simulink library "halout"  (R2021b)
settings: Solver=VariableStepAuto  StartTime=0.0  StopTime=10.0  RelTol=1e-3
undefined symbols (not defined in the file): C_TASK_5MS_S, FALSE, KHAL_CAN1FD1APS3E2E_flg, KHAL_CAN1FD1APS3TxReq_flg, KHAL_CAN1FD1VCU2E2E_flg, KHAL_CAN1FD1VCU2TxReq_flg, KHAL_CAN1FD1VCU3E2E_flg, KHAL_CAN1FD1VCU3TxReq_flg, KHAL_CAN1TxReq_flg, KHAL_CAN1VMCFCM1E2E_flg, KHAL_CAN1VMCFCM1TxReq_flg, KHAL_CAN2TxReq_flg, KHAL_CAN3FD3VCU1toNIDECTxReq_flg, KHAL_CAN3FD3VCU1TxReq_flg, KHAL_CAN3FD3VCU2E2E_flg, KHAL_CAN3FD3VCU2toNIDECE2E_flg, KHAL_CAN3FD3VCU2toNIDECTxReq_flg, KHAL_CAN3FD3VCU2TxReq_flg, KHAL_CAN3TxReq_flg, KHAL_CAN4FD4CE1000E2E_flg, KHAL_CAN4FD4CE1000TxReq_flg, KHAL_CAN4TxReq_flg, KHAL_CAN5TxReq_flg, KHAL_CAN6FD6APS3E2E_flg, KHAL_CAN6FD6APS3TxReq_flg, KHAL_CAN6FD6VCU2E2E_flg, KHAL_CAN6FD6VCU2TxReq_flg, KHAL_CAN6TxReq_flg, ONE_INT, TRUE, ZERO_INT
libraries: FVT_lib x549, simulink x244
(part 15 of 27)

== system halout/HAL_OUT/CAN1/FD1_APS3_0x238/Byte_9 ==
  FDC_APS_Active_Sta : Inport
  FDC_APS_SpeedReq_Cmd : Inport  Port=2
  FDC_APS_VMCReqA_Cmd : Inport  Port=3
  FDC_RAPS_ErrLv1_Flg : Inport  Port=4
  FDC_VCU_RAPSErrLv2_Flg : Inport  Port=5
  BitwiseOR : simulink/Logic and Bit Operations/Bitwise Operator  logicop=OR  UseBitMask=off  NumInputPorts=5  BitMask=bin2dec('11011001')  BitMaskRealWorld=Stored Integer
  SignalPack : FVT_lib/hal/SignalPack  RightShiftCnt=0  BitMask=2^1-1  LeftShiftCnt=4
  SignalPack1 : FVT_lib/hal/SignalPack  RightShiftCnt=8  BitMask=2^4-1  LeftShiftCnt=0
  SignalPack2 : FVT_lib/hal/SignalPack  RightShiftCnt=0  BitMask=2^1-1  LeftShiftCnt=5
  SignalPack3 : FVT_lib/hal/SignalPack  RightShiftCnt=0  BitMask=2^1-1  LeftShiftCnt=6
  SignalPack4 : FVT_lib/hal/SignalPack  RightShiftCnt=0  BitMask=2^1-1  LeftShiftCnt=7
  UnitConverter{,1..2,4..9} (9 alike) : DataTypeConversion  OutDataTypeStr=uint8  RndMeth=Round
  UnitConverter3 : DataTypeConversion  OutDataTypeStr=uint16  RndMeth=Round
  convert_out : FVT_lib/hal/convert_out  gain=0.125  offset=0
  Byte_9 : Outport
  wires:
  BitwiseOR/1 -> Byte_9/1
  UnitConverter/1 -> BitwiseOR/1
  SignalPack/1 -> UnitConverter/1
  UnitConverter1/1 -> SignalPack/1
  FDC_APS_Active_Sta/1 -> UnitConverter1/1
  UnitConverter2/1 -> BitwiseOR/2
  SignalPack1/1 -> UnitConverter2/1
  UnitConverter3/1 -> SignalPack1/1
  convert_out/1 -> UnitConverter3/1
  FDC_APS_SpeedReq_Cmd/1 -> convert_out/1
  UnitConverter4/1 -> BitwiseOR/3
  SignalPack2/1 -> UnitConverter4/1
  UnitConverter5/1 -> SignalPack2/1
  FDC_APS_VMCReqA_Cmd/1 -> UnitConverter5/1
  UnitConverter6/1 -> BitwiseOR/4
  SignalPack3/1 -> UnitConverter6/1
  UnitConverter7/1 -> SignalPack3/1
  FDC_RAPS_ErrLv1_Flg/1 -> UnitConverter7/1
  UnitConverter8/1 -> BitwiseOR/5
  SignalPack4/1 -> UnitConverter8/1
  UnitConverter9/1 -> SignalPack4/1
  FDC_VCU_RAPSErrLv2_Flg/1 -> UnitConverter9/1

== system halout/HAL_OUT/CAN1/FD1_APS3_0x238/CAASSta ==
  CAASSta : Inport
  Data Type Conversion : DataTypeConversion  OutDataTypeStr=uint8  RndMeth=Round
  CAN1_CAAS_Sta : Outport
  wires:
  Data Type Conversion/1 -> CAN1_CAAS_Sta/1
  CAASSta/1 -> Data Type Conversion/1

== system halout/HAL_OUT/CAN1/FD1_APS3_0x238/CRC8_IfAction_Tx ==
  CAN_E2E_flg : Inport
  DataID1 : Inport  Port=2
  DataID2 : Inport  Port=3
  RawData : Inport  Port=4
  Data Type Conversion : DataTypeConversion  OutDataTypeStr=uint8
  If : If
  If Action Subsystem : Subsystem  TreatAsAtomicUnit=on
  If Action Subsystem1 : Subsystem  TreatAsAtomicUnit=on
  Merge : Merge
  CRC8 : Outport
  wires:
  If/2 -> If Action Subsystem/Action
  If/1 -> If Action Subsystem1/Action
  CAN_E2E_flg/1 -> [CAN_E2E_flg]
  DataID1/1 -> [DataID1]
  DataID2/1 -> [DataID2]
  RawData/1 -> [RawData]
  [CAN_E2E_flg] -> Data Type Conversion/1
  [DataID1] -> If Action Subsystem1/1(CAN_E2E_ID1)
  [DataID2] -> If Action Subsystem1/2(CAN_E2E_ID2)
  [RawData] -> If Action Subsystem1/3(Byte1)
  [RawData] -> If Action Subsystem/1(Byte1)
  If Action Subsystem1/1(CRC8_E2EResult) -> Merge/1
  If Action Subsystem/1(CRC8_Result) -> Merge/2
  Merge/1 -> CRC8/1
  Data Type Conversion/1 -> If/1

== system halout/HAL_OUT/CAN1/FD1_APS3_0x238/FDCAPSActiveSta ==
  FDCAPSActiveSta : Inport
  Data Type Conversion : DataTypeConversion  OutDataTypeStr=uint8  RndMeth=Round
  CAN1_FDC_APS_Active_Sta : Outport
  wires:
  Data Type Conversion/1 -> CAN1_FDC_APS_Active_Sta/1
  FDCAPSActiveSta/1 -> Data Type Conversion/1

== system halout/HAL_OUT/CAN1/FD1_APS3_0x238/FDCAPSCaasActiveSta ==
  FDCAPSCaasActiveSta : Inport
  Data Type Conversion : DataTypeConversion  OutDataTypeStr=uint8  RndMeth=Round
  CAN1_FDC_APS_CaasActive_Sta : Outport
  wires:
  Data Type Conversion/1 -> CAN1_FDC_APS_CaasActive_Sta/1
  FDCAPSCaasActiveSta/1 -> Data Type Conversion/1

== system halout/HAL_OUT/CAN1/FD1_APS3_0x238/FDCAPSCaasCtrlAvailSta ==
  FDCAPSCaasCtrlAvailSta : Inport
  Data Type Conversion : DataTypeConversion  OutDataTypeStr=uint8  RndMeth=Round
  CAN1_FDC_APS_CaasCtrlAvail_Sta : Outport
  wires:
  Data Type Conversion/1 -> CAN1_FDC_APS_CaasCtrlAvail_Sta/1
  FDCAPSCaasCtrlAvailSta/1 -> Data Type Conversion/1

== system halout/HAL_OUT/CAN1/FD1_APS3_0x238/FDCAPSCaasVMCReqACmd ==
  FDCAPSCaasVMCReqACmd : Inport
  Data Type Conversion : DataTypeConversion  OutDataTypeStr=uint8  RndMeth=Round
  CAN1_FDC_APS_CaasVMCReqA_Cmd : Outport
  wires:
  Data Type Conversion/1 -> CAN1_FDC_APS_CaasVMCReqA_Cmd/1
  FDCAPSCaasVMCReqACmd/1 -> Data Type Conversion/1

== system halout/HAL_OUT/CAN1/FD1_APS3_0x238/FDCAPSCtrlAvailSta ==
  FDCAPSCtrlAvailSta : Inport
  Data Type Conversion : DataTypeConversion  OutDataTypeStr=uint8  RndMeth=Round
  CAN1_FDC_APS_CtrlAvail_Sta : Outport
  wires:
  Data Type Conversion/1 -> CAN1_FDC_APS_CtrlAvail_Sta/1
  FDCAPSCtrlAvailSta/1 -> Data Type Conversion/1

== system halout/HAL_OUT/CAN1/FD1_APS3_0x238/FDCAPSShftPosnReqCmd ==
  FDCAPSShftPosnReqCmd : Inport
  Data Type Conversion : DataTypeConversion  OutDataTypeStr=uint8  RndMeth=Round
  CAN1_FDC_APS_ShftPosnReq_Cmd : Outport
  wires:
  Data Type Conversion/1 -> CAN1_FDC_APS_ShftPosnReq_Cmd/1
  FDCAPSShftPosnReqCmd/1 -> Data Type Conversion/1

== system halout/HAL_OUT/CAN1/FD1_APS3_0x238/FDCAPSSpeedReqCmd ==
  FDCAPSSpeedReqCmd : Inport
  Data Type Conversion : DataTypeConversion  OutDataTypeStr=uint16  RndMeth=Round
  convert_out : FVT_lib/hal/convert_out  gain=0.125  offset=0
  CAN1_FDC_APS_SpeedReq_Cmd : Outport
  wires:
  Data Type Conversion/1 -> CAN1_FDC_APS_SpeedReq_Cmd/1
  convert_out/1 -> Data Type Conversion/1
  FDCAPSSpeedReqCmd/1 -> convert_out/1

== system halout/HAL_OUT/CAN1/FD1_APS3_0x238/FDCAPSVMCReqACmd ==
  FDCAPSVMCReqACmd : Inport
  Data Type Conversion : DataTypeConversion  OutDataTypeStr=uint8  RndMeth=Round
  CAN1_FDC_APS_VMCReqA_Cmd : Outport
  wires:
  Data Type Conversion/1 -> CAN1_FDC_APS_VMCReqA_Cmd/1
  FDCAPSVMCReqACmd/1 -> Data Type Conversion/1

== system halout/HAL_OUT/CAN1/FD1_APS3_0x238/FDCRAPSBCMLampCmd ==
  FDCRAPSBCMLampCmd : Inport
  Data Type Conversion : DataTypeConversion  OutDataTypeStr=uint8  RndMeth=Round
  CAN1_FDC_RAPS_BCMLamp_Cmd : Outport
  wires:
  Data Type Conversion/1 -> CAN1_FDC_RAPS_BCMLamp_Cmd/1
  FDCRAPSBCMLampCmd/1 -> Data Type Conversion/1

== system halout/HAL_OUT/CAN1/FD1_APS3_0x238/FDCRAPSBCMLockReqCmd ==
  FDCRAPSBCMLockReqCmd : Inport
  Data Type Conversion : DataTypeConversion  OutDataTypeStr=uint8  RndMeth=Round
  CAN1_FDC_RAPS_BCMLockReq_Cmd : Outport
  wires:
  Data Type Conversion/1 -> CAN1_FDC_RAPS_BCMLockReq_Cmd/1
  FDCRAPSBCMLockReqCmd/1 -> Data Type Conversion/1

== system halout/HAL_OUT/CAN1/FD1_APS3_0x238/FDCRAPSErrLv1Flg ==
  FDCRAPSErrLv1Flg : Inport
  Data Type Conversion : DataTypeConversion  OutDataTypeStr=uint8  RndMeth=Round
  CAN1_FDC_RAPS_ErrLv1_Flg : Outport
  wires:
  Data Type Conversion/1 -> CAN1_FDC_RAPS_ErrLv1_Flg/1
  FDCRAPSErrLv1Flg/1 -> Data Type Conversion/1

== system halout/HAL_OUT/CAN1/FD1_APS3_0x238/FDCRAPSPwrReqAvailSta ==
  FDCRAPSPwrReqAvailSta : Inport
  Data Type Conversion : DataTypeConversion  OutDataTypeStr=uint8  RndMeth=Round
  CAN1_FDC_RAPS_PwrReqAvail_Sta : Outport
  wires:
  Data Type Conversion/1 -> CAN1_FDC_RAPS_PwrReqAvail_Sta/1
  FDCRAPSPwrReqAvailSta/1 -> Data Type Conversion/1

== system halout/HAL_OUT/CAN1/FD1_APS3_0x238/FDCRAPSPwrReqCmd ==
  FDCRAPSPwrReqCmd : Inport
  Data Type Conversion : DataTypeConversion  OutDataTypeStr=uint8  RndMeth=Round
  CAN1_FDC_RAPS_PwrReq_Cmd : Outport
  wires:
  Data Type Conversion/1 -> CAN1_FDC_RAPS_PwrReq_Cmd/1
  FDCRAPSPwrReqCmd/1 -> Data Type Conversion/1

== system halout/HAL_OUT/CAN1/FD1_APS3_0x238/FDCVCURAPSErrLv2Flg ==
  FDCVCURAPSErrLv2Flg : Inport
  Data Type Conversion : DataTypeConversion  OutDataTypeStr=uint8  RndMeth=Round
  CAN1_FDC_VCU_RAPSErrLv2_Flg : Outport
  wires:
  Data Type Conversion/1 -> CAN1_FDC_VCU_RAPSErrLv2_Flg/1
  FDCVCURAPSErrLv2Flg/1 -> Data Type Conversion/1

== system halout/HAL_OUT/CAN1/FD1_APS3_0x238/FDCVCURAPSErrLv3Flg ==
  FDCVCURAPSErrLv3Flg : Inport
  Data Type Conversion : DataTypeConversion  OutDataTypeStr=uint8  RndMeth=Round
  CAN1_FDC_VCU_RAPSErrLv3_Flg : Outport
  wires:
  Data Type Conversion/1 -> CAN1_FDC_VCU_RAPSErrLv3_Flg/1
  FDCVCURAPSErrLv3Flg/1 -> Data Type Conversion/1

== system halout/HAL_OUT/CAN1/FD1_APS3_0x238/FDCVMCAPSAngleTarget ==
  FDCVMCAPSAngleTarget : Inport
  Data Type Conversion : DataTypeConversion  OutDataTypeStr=uint16  RndMeth=Round
  convert_out : FVT_lib/hal/convert_out  gain=0.1  offset=-900
  CAN1_FDC_VMC_APS_Angle_Target : Outport
  wires:
  Data Type Conversion/1 -> CAN1_FDC_VMC_APS_Angle_Target/1
  convert_out/1 -> Data Type Conversion/1
  FDCVMCAPSAngleTarget/1 -> convert_out/1

== system halout/HAL_OUT/CAN1/FD1_APS3_0x238/FDCVMCAPSRqEPSCtrl ==
  FDCVMCAPSRqEPSCtrl : Inport
  Data Type Conversion : DataTypeConversion  OutDataTypeStr=uint8  RndMeth=Round
  CAN1_FDC_VMC_APS_Rq_EPS_Ctrl : Outport
  wires:
  Data Type Conversion/1 -> CAN1_FDC_VMC_APS_Rq_EPS_Ctrl/1
  FDCVMCAPSRqEPSCtrl/1 -> Data Type Conversion/1

== system halout/HAL_OUT/CAN1/FD1_APS3_0x238/FDCVMCAPSVRqEPSCtrl ==
  FDCVMCAPSVRqEPSCtrl : Inport
  Data Type Conversion : DataTypeConversion  OutDataTypeStr=uint8  RndMeth=Round
  CAN1_FDC_VMC_APS_V_Rq_EPS_Ctrl : Outport
  wires:
  Data Type Conversion/1 -> CAN1_FDC_VMC_APS_V_Rq_EPS_Ctrl/1
  FDCVMCAPSVRqEPSCtrl/1 -> Data Type Conversion/1

== system halout/HAL_OUT/CAN1/FD1_APS3_0x238/SPTGDet ==
  SPTGDet : Inport
  Data Type Conversion : DataTypeConversion  OutDataTypeStr=uint8  RndMeth=Round
  CAN1_SPTGDet : Outport
  wires:
  Data Type Conversion/1 -> CAN1_SPTGDet/1
  SPTGDet/1 -> Data Type Conversion/1

== system halout/HAL_OUT/CAN1/FD1_APS3_0x238/SPTGSta ==
  SPTGSta : Inport
  Data Type Conversion : DataTypeConversion  OutDataTypeStr=uint8  RndMeth=Round
  CAN1_SPTG_Sta : Outport
  wires:
  Data Type Conversion/1 -> CAN1_SPTG_Sta/1
  SPTGSta/1 -> Data Type Conversion/1

== system halout/HAL_OUT/CAN1/FD1_BCM1_0x216/AllDoorSW ==
  AllDoorSW : Inport
  Data Type Conversion : DataTypeConversion  OutDataTypeStr=uint8  RndMeth=Round
  CAN1_AllDoorSW : Outport
  wires:
  Data Type Conversion/1 -> CAN1_AllDoorSW/1
  AllDoorSW/1 -> Data Type Conversion/1

== system halout/HAL_OUT/CAN1/FD1_BCM1_0x216/AntiTheftSeatFold ==
  AntiTheftSeatFold : Inport
  Data Type Conversion : DataTypeConversion  OutDataTypeStr=uint8  RndMeth=Round
  CAN1_AntiTheftSeatFold : Outport
  wires:
  Data Type Conversion/1 -> CAN1_AntiTheftSeatFold/1
  AntiTheftSeatFold/1 -> Data Type Conversion/1

== system halout/HAL_OUT/CAN1/FD1_BCM1_0x216/AntitheftSta ==
  AntitheftSta : Inport
  Data Type Conversion : DataTypeConversion  OutDataTypeStr=uint8  RndMeth=Round
  CAN1_AntitheftSta : Outport
  wires:
  Data Type Conversion/1 -> CAN1_AntitheftSta/1
  AntitheftSta/1 -> Data Type Conversion/1

== system halout/HAL_OUT/CAN1/FD1_BCM1_0x216/BCMBuzzerReq ==
  BCMBuzzerReq : Inport
  Data Type Conversion : DataTypeConversion  OutDataTypeStr=uint8  RndMeth=Round
  CAN1_BCM_Buzzer_Req : Outport
  wires:
  Data Type Conversion/1 -> CAN1_BCM_Buzzer_Req/1
  BCMBuzzerReq/1 -> Data Type Conversion/1

== system halout/HAL_OUT/CAN1/FD1_BCM1_0x216/BCMDoorLockSta ==
  BCMDoorLockSta : Inport
  Data Type Conversion : DataTypeConversion  OutDataTypeStr=uint8  RndMeth=Round
  CAN1_BCM_DoorLock_Sta : Outport
  wires:
  Data Type Conversion/1 -> CAN1_BCM_DoorLock_Sta/1
  BCMDoorLockSta/1 -> Data Type Conversion/1

== system halout/HAL_OUT/CAN1/FD1_BCM1_0x216/BrakeLamp ==
  BrakeLamp : Inport
  Data Type Conversion : DataTypeConversion  OutDataTypeStr=uint8  RndMeth=Round
  CAN1_BrakeLamp : Outport
  wires:
  Data Type Conversion/1 -> CAN1_BrakeLamp/1
  BrakeLamp/1 -> Data Type Conversion/1

== system halout/HAL_OUT/CAN1/FD1_BCM1_0x216/CTDCtrl ==
  CTDCtrl : Inport
  Data Type Conversion : DataTypeConversion  OutDataTypeStr=uint8  RndMeth=Round
  CAN1_CTDCtrl : Outport
  wires:
  Data Type Conversion/1 -> CAN1_CTDCtrl/1
  CTDCtrl/1 -> Data Type Conversion/1

== system halout/HAL_OUT/CAN1/FD1_BCM1_0x216/CTDLockSW ==
  CTDLockSW : Inport
  Data Type Conversion : DataTypeConversion  OutDataTypeStr=uint8  RndMeth=Round
  CAN1_CTDLockSW : Outport
  wires:
  Data Type Conversion/1 -> CAN1_CTDLockSW/1
  CTDLockSW/1 -> Data Type Conversion/1

== system halout/HAL_OUT/CAN1/FD1_BCM1_0x216/CTDUnlockSW ==
  CTDUnlockSW : Inport
  Data Type Conversion : DataTypeConversion  OutDataTypeStr=uint8  RndMeth=Round
  CAN1_CTDUnlockSW : Outport
  wires:
  Data Type Conversion/1 -> CAN1_CTDUnlockSW/1
  CTDUnlockSW/1 -> Data Type Conversion/1

== system halout/HAL_OUT/CAN1/FD1_BCM1_0x216/CrashDetd ==
  CrashDetd : Inport
  Data Type Conversion : DataTypeConversion  OutDataTypeStr=uint8  RndMeth=Round
  CAN1_CrashDetd : Outport
  wires:
  Data Type Conversion/1 -> CAN1_CrashDetd/1
  CrashDetd/1 -> Data Type Conversion/1

== system halout/HAL_OUT/CAN1/FD1_BCM1_0x216/Dimmer ==
  Dimmer : Inport
  Data Type Conversion : DataTypeConversion  OutDataTypeStr=uint8  RndMeth=Round
  CAN1_Dimmer : Outport
  wires:
  Data Type Conversion/1 -> CAN1_Dimmer/1
  Dimmer/1 -> Data Type Conversion/1

== system halout/HAL_OUT/CAN1/FD1_BCM1_0x216/DimmerEN ==
  DimmerEN : Inport
  Data Type Conversion : DataTypeConversion  OutDataTypeStr=uint8  RndMeth=Round
  CAN1_DimmerEN : Outport
  wires:
  Data Type Conversion/1 -> CAN1_DimmerEN/1
  DimmerEN/1 -> Data Type Conversion/1

== system halout/HAL_OUT/CAN1/FD1_BCM1_0x216/DoorLockIND ==
  DoorLockIND : Inport
  Data Type Conversion : DataTypeConversion  OutDataTypeStr=uint8  RndMeth=Round
  CAN1_DoorLockIND : Outport
  wires:
  Data Type Conversion/1 -> CAN1_DoorLockIND/1
  DoorLockIND/1 -> Data Type Conversion/1

== system halout/HAL_OUT/CAN1/FD1_BCM1_0x216/DrDoorSW ==
  DrDoorSW : Inport
  Data Type Conversion : DataTypeConversion  OutDataTypeStr=uint8  RndMeth=Round
  CAN1_DrDoorSW : Outport
  wires:
  Data Type Conversion/1 -> CAN1_DrDoorSW/1
  DrDoorSW/1 -> Data Type Conversion/1

== system halout/HAL_OUT/CAN1/FD1_BCM1_0x216/FrChargingDoorCtrl ==
  FrChargingDoorCtrl : Inport
  Data Type Conversion : DataTypeConversion  OutDataTypeStr=uint8  RndMeth=Round
  CAN1_Fr_ChargingDoorCtrl : Outport
  wires:
  Data Type Conversion/1 -> CAN1_Fr_ChargingDoorCtrl/1
  FrChargingDoorCtrl/1 -> Data Type Conversion/1

== system halout/HAL_OUT/CAN1/FD1_BCM1_0x216/FrFogLamp ==
  FrFogLamp : Inport
  Data Type Conversion : DataTypeConversion  OutDataTypeStr=uint8  RndMeth=Round
  CAN1_Fr_FogLamp : Outport
  wires:
  Data Type Conversion/1 -> CAN1_Fr_FogLamp/1
  FrFogLamp/1 -> Data Type Conversion/1

== system halout/HAL_OUT/CAN1/FD1_BCM1_0x216/FrWiperH ==
  FrWiperH : Inport
  Data Type Conversion : DataTypeConversion  OutDataTypeStr=uint8  RndMeth=Round
  CAN1_Fr_Wiper_H : Outport
  wires:
  Data Type Conversion/1 -> CAN1_Fr_Wiper_H/1
  FrWiperH/1 -> Data Type Conversion/1

== system halout/HAL_OUT/CAN1/FD1_BCM1_0x216/FrWiperL ==
  FrWiperL : Inport
  Data Type Conversion : DataTypeConversion  OutDataTypeStr=uint8  RndMeth=Round
  CAN1_Fr_Wiper_L : Outport
  wires:
  Data Type Conversion/1 -> CAN1_Fr_Wiper_L/1
  FrWiperL/1 -> Data Type Conversion/1

== system halout/HAL_OUT/CAN1/FD1_BCM1_0x216/HBeam ==
  HBeam : Inport
  Data Type Conversion : DataTypeConversion  OutDataTypeStr=uint8  RndMeth=Round
  CAN1_H_Beam : Outport
  wires:
  Data Type Conversion/1 -> CAN1_H_Beam/1
  HBeam/1 -> Data Type Conversion/1

== system halout/HAL_OUT/CAN1/FD1_BCM1_0x216/HazardSW ==
  HazardSW : Inport
  Data Type Conversion : DataTypeConversion  OutDataTypeStr=uint8  RndMeth=Round
  CAN1_HazardSW : Outport
  wires:
  Data Type Conversion/1 -> CAN1_HazardSW/1
  HazardSW/1 -> Data Type Conversion/1

== system halout/HAL_OUT/CAN1/FD1_BCM1_0x216/HoodSW ==
  HoodSW : Inport
  Data Type Conversion : DataTypeConversion  OutDataTypeStr=uint8  RndMeth=Round
  CAN1_HoodSW : Outport
  wires:
  Data Type Conversion/1 -> CAN1_HoodSW/1
  HoodSW/1 -> Data Type Conversion/1

== system halout/HAL_OUT/CAN1/FD1_BCM1_0x216/HornCtrl ==
  HornCtrl : Inport
  Data Type Conversion : DataTypeConversion  OutDataTypeStr=uint8  RndMeth=Round
  CAN1_HornCtrl : Outport
  wires:
  Data Type Conversion/1 -> CAN1_HornCtrl/1
  HornCtrl/1 -> Data Type Conversion/1

== system halout/HAL_OUT/CAN1/FD1_BCM1_0x216/LAPMWdwEnable ==
  LAPMWdwEnable : Inport
  Data Type Conversion : DataTypeConversion  OutDataTypeStr=uint8  RndMeth=Round
  CAN1_L_APM_WdwEnable : Outport
  wires:
  Data Type Conversion/1 -> CAN1_L_APM_WdwEnable/1
  LAPMWdwEnable/1 -> Data Type Conversion/1

== system halout/HAL_OUT/CAN1/FD1_BCM1_0x216/LBSD ==
  LBSD : Inport
  Data Type Conversion : DataTypeConversion  OutDataTypeStr=uint8  RndMeth=Round
  CAN1_LBSD : Outport
  wires:
  Data Type Conversion/1 -> CAN1_LBSD/1
  LBSD/1 -> Data Type Conversion/1

== system halout/HAL_OUT/CAN1/FD1_BCM1_0x216/LBeam ==
  LBeam : Inport
  Data Type Conversion : DataTypeConversion  OutDataTypeStr=uint8  RndMeth=Round
  CAN1_L_Beam : Outport
  wires:
  Data Type Conversion/1 -> CAN1_L_Beam/1
  LBeam/1 -> Data Type Conversion/1

== system halout/HAL_OUT/CAN1/FD1_BCM1_0x216/LDRL ==
  LDRL : Inport
  Data Type Conversion : DataTypeConversion  OutDataTypeStr=uint8  RndMeth=Round
  CAN1_LDRL : Outport
  wires:
  Data Type Conversion/1 -> CAN1_LDRL/1
  LDRL/1 -> Data Type Conversion/1

== system halout/HAL_OUT/CAN1/FD1_BCM1_0x216/LTurnLP ==
  LTurnLP : Inport
  Data Type Conversion : DataTypeConversion  OutDataTypeStr=uint8  RndMeth=Round
  CAN1_LTurnLP : Outport
  wires:
  Data Type Conversion/1 -> CAN1_LTurnLP/1
  LTurnLP/1 -> Data Type Conversion/1

== system halout/HAL_OUT/CAN1/FD1_BCM1_0x216/LockSetting ==
  LockSetting : Inport
  Data Type Conversion : DataTypeConversion  OutDataTypeStr=uint8  RndMeth=Round
  CAN1_LockSetting : Outport
  wires:
  Data Type Conversion/1 -> CAN1_LockSetting/1
  LockSetting/1 -> Data Type Conversion/1

== system halout/HAL_OUT/CAN1/FD1_BCM1_0x216/MirrorCtrl ==
  MirrorCtrl : Inport
  Data Type Conversion : DataTypeConversion  OutDataTypeStr=uint8  RndMeth=Round
  CAN1_MirrorCtrl : Outport
  wires:
  Data Type Conversion/1 -> CAN1_MirrorCtrl/1
  MirrorCtrl/1 -> Data Type Conversion/1

== system halout/HAL_OUT/CAN1/FD1_BCM1_0x216/MirrorDefog ==
  MirrorDefog : Inport
  Data Type Conversion : DataTypeConversion  OutDataTypeStr=uint8  RndMeth=Round
  CAN1_MirrorDefog : Outport
  wires:
  Data Type Conversion/1 -> CAN1_MirrorDefog/1
  MirrorDefog/1 -> Data Type Conversion/1

== system halout/HAL_OUT/CAN1/FD1_BCM1_0x216/PosLamp ==
  PosLamp : Inport
  Data Type Conversion : DataTypeConversion  OutDataTypeStr=uint8  RndMeth=Round
  CAN1_PosLamp : Outport
  wires:
  Data Type Conversion/1 -> CAN1_PosLamp/1
  PosLamp/1 -> Data Type Conversion/1

== system halout/HAL_OUT/CAN1/FD1_BCM1_0x216/PsDoorSW ==
  PsDoorSW : Inport
  Data Type Conversion : DataTypeConversion  OutDataTypeStr=uint8  RndMeth=Round
  CAN1_PsDoorSW : Outport
  wires:
  Data Type Conversion/1 -> CAN1_PsDoorSW/1
  PsDoorSW/1 -> Data Type Conversion/1

== system halout/HAL_OUT/CAN1/FD1_BCM1_0x216/RBSD ==
  RBSD : Inport
  Data Type Conversion : DataTypeConversion  OutDataTypeStr=uint8  RndMeth=Round
  CAN1_RBSD : Outport
  wires:
  Data Type Conversion/1 -> CAN1_RBSD/1
  RBSD/1 -> Data Type Conversion/1

== system halout/HAL_OUT/CAN1/FD1_BCM1_0x216/RDRL ==
  RDRL : Inport
  Data Type Conversion : DataTypeConversion  OutDataTypeStr=uint8  RndMeth=Round
  CAN1_RDRL : Outport
  wires:
  Data Type Conversion/1 -> CAN1_RDRL/1
  RDRL/1 -> Data Type Conversion/1

== system halout/HAL_OUT/CAN1/FD1_BCM1_0x216/RLDoorSW ==
  RLDoorSW : Inport
  Data Type Conversion : DataTypeConversion  OutDataTypeStr=uint8  RndMeth=Round
  CAN1_RLDoorSW : Outport
  wires:
  Data Type Conversion/1 -> CAN1_RLDoorSW/1
  RLDoorSW/1 -> Data Type Conversion/1

== system halout/HAL_OUT/CAN1/FD1_BCM1_0x216/RRDoorSW ==
  RRDoorSW : Inport
  Data Type Conversion : DataTypeConversion  OutDataTypeStr=uint8  RndMeth=Round
  CAN1_RRDoorSW : Outport
  wires:
  Data Type Conversion/1 -> CAN1_RRDoorSW/1
  RRDoorSW/1 -> Data Type Conversion/1

== system halout/HAL_OUT/CAN1/FD1_BCM1_0x216/RTurnLP ==
  RTurnLP : Inport
  Data Type Conversion : DataTypeConversion  OutDataTypeStr=uint8  RndMeth=Round
  CAN1_RTurnLP : Outport
  wires:
  Data Type Conversion/1 -> CAN1_RTurnLP/1
  RTurnLP/1 -> Data Type Conversion/1

== system halout/HAL_OUT/CAN1/FD1_BCM1_0x216/ReverseLamp ==
  ReverseLamp : Inport
  Data Type Conversion : DataTypeConversion  OutDataTypeStr=uint8  RndMeth=Round
  CAN1_ReverseLamp : Outport
  wires:
  Data Type Conversion/1 -> CAN1_ReverseLamp/1
  ReverseLamp/1 -> Data Type Conversion/1

== system halout/HAL_OUT/CAN1/FD1_BCM1_0x216/RoomLampH ==
  RoomLampH : Inport
  Data Type Conversion : DataTypeConversion  OutDataTypeStr=uint8  RndMeth=Round
  CAN1_RoomLampH : Outport
  wires:
  Data Type Conversion/1 -> CAN1_RoomLampH/1
  RoomLampH/1 -> Data Type Conversion/1

== system halout/HAL_OUT/CAN1/FD1_BCM1_0x216/RoomLampL ==
  RoomLampL : Inport
  Data Type Conversion : DataTypeConversion  OutDataTypeStr=uint8  RndMeth=Round
  CAN1_RoomLampL : Outport
  wires:
  Data Type Conversion/1 -> CAN1_RoomLampL/1
  RoomLampL/1 -> Data Type Conversion/1

== system halout/HAL_OUT/CAN1/FD1_BCM1_0x216/RrChargingDoorCtrl ==
  RrChargingDoorCtrl : Inport
  Data Type Conversion : DataTypeConversion  OutDataTypeStr=uint8  RndMeth=Round
  CAN1_Rr_ChargingDoorCtrl : Outport
  wires:
  Data Type Conversion/1 -> CAN1_Rr_ChargingDoorCtrl/1
  RrChargingDoorCtrl/1 -> Data Type Conversion/1

== system halout/HAL_OUT/CAN1/FD1_BCM1_0x216/RrDefog ==
  RrDefog : Inport
  Data Type Conversion : DataTypeConversion  OutDataTypeStr=uint8  RndMeth=Round
  CAN1_Rr_Defog : Outport
  wires:
  Data Type Conversion/1 -> CAN1_Rr_Defog/1
  RrDefog/1 -> Data Type Conversion/1

== system halout/HAL_OUT/CAN1/FD1_BCM1_0x216/RrFogLamp ==
  RrFogLamp : Inport
  Data Type Conversion : DataTypeConversion  OutDataTypeStr=uint8  RndMeth=Round
  CAN1_Rr_FogLamp : Outport
  wires:
  Data Type Conversion/1 -> CAN1_Rr_FogLamp/1
  RrFogLamp/1 -> Data Type Conversion/1

== system halout/HAL_OUT/CAN1/FD1_BCM1_0x216/RrWiper ==
  RrWiper : Inport
  Data Type Conversion : DataTypeConversion  OutDataTypeStr=uint8  RndMeth=Round
  CAN1_Rr_Wiper : Outport
  wires:
  Data Type Conversion/1 -> CAN1_Rr_Wiper/1
  RrWiper/1 -> Data Type Conversion/1

== system halout/HAL_OUT/CAN1/FD1_BCM1_0x216/TailgateHDSW ==
  TailgateHDSW : Inport
  Data Type Conversion : DataTypeConversion  OutDataTypeStr=uint8  RndMeth=Round
  CAN1_TailgateHDSW : Outport
  wires:
  Data Type Conversion/1 -> CAN1_TailgateHDSW/1
  TailgateHDSW/1 -> Data Type Conversion/1

== system halout/HAL_OUT/CAN1/FD1_BCM1_0x216/TailgateRemote ==
  TailgateRemote : Inport
  Data Type Conversion : DataTypeConversion  OutDataTypeStr=uint8  RndMeth=Round
  CAN1_TailgateRemote : Outport
  wires:
  Data Type Conversion/1 -> CAN1_TailgateRemote/1
  TailgateRemote/1 -> Data Type Conversion/1

== system halout/HAL_OUT/CAN1/FD1_BCM1_0x216/TailgateSW ==
  TailgateSW : Inport
  Data Type Conversion : DataTypeConversion  OutDataTypeStr=uint8  RndMeth=Round
  CAN1_Tailgate_SW : Outport
  wires:
  Data Type Conversion/1 -> CAN1_Tailgate_SW/1
  TailgateSW/1 -> Data Type Conversion/1

== system halout/HAL_OUT/CAN1/FD1_BCM1_0x216/TrunkRel ==
  TrunkRel : Inport
  Data Type Conversion : DataTypeConversion  OutDataTypeStr=uint8  RndMeth=Round
  CAN1_TrunkRel : Outport
  wires:
  Data Type Conversion/1 -> CAN1_TrunkRel/1
  TrunkRel/1 -> Data Type Conversion/1

== system halout/HAL_OUT/CAN1/FD1_BCM1_0x216/WasherCtrl ==
  WasherCtrl : Inport
  Data Type Conversion : DataTypeConversion  OutDataTypeStr=uint8  RndMeth=Round
  CAN1_WasherCtrl : Outport
  wires:
  Data Type Conversion/1 -> CAN1_WasherCtrl/1
  WasherCtrl/1 -> Data Type Conversion/1

== system halout/HAL_OUT/CAN1/FD1_BCM1_0x216/WiperFixMode ==
  WiperFixMode : Inport
  Data Type Conversion : DataTypeConversion  OutDataTypeStr=uint8  RndMeth=Round
  CAN1_WiperFixMode : Outport
  wires:
  Data Type Conversion/1 -> CAN1_WiperFixMode/1
  WiperFixMode/1 -> Data Type Conversion/1

== system halout/HAL_OUT/CAN1/FD1_THCM1_0x182/BatteryMode ==
  BatteryMode : Inport
  Data Type Conversion : DataTypeConversion  OutDataTypeStr=uint8  RndMeth=Round
  CAN1_BatteryMode : Outport
  wires:
  Data Type Conversion/1 -> CAN1_BatteryMode/1
  BatteryMode/1 -> Data Type Conversion/1

== system halout/HAL_OUT/CAN1/FD1_THCM1_0x182/CCUACLampSts ==
  CCUACLampSts : Inport
  Data Type Conversion : DataTypeConversion  OutDataTypeStr=uint8  RndMeth=Round
  CAN1_CCU_ACLampSts : Outport
  wires:
  Data Type Conversion/1 -> CAN1_CCU_ACLampSts/1
  CCUACLampSts/1 -> Data Type Conversion/1

== system halout/HAL_OUT/CAN1/FD1_THCM1_0x182/CCUACMaxLampSts ==
  CCUACMaxLampSts : Inport
  Data Type Conversion : DataTypeConversion  OutDataTypeStr=uint8  RndMeth=Round
  CAN1_CCU_ACMaxLampSts : Outport
  wires:
  Data Type Conversion/1 -> CAN1_CCU_ACMaxLampSts/1
  CCUACMaxLampSts/1 -> Data Type Conversion/1

== system halout/HAL_OUT/CAN1/FD1_THCM1_0x182/CCUAutoLampSts ==
  CCUAutoLampSts : Inport
  Data Type Conversion : DataTypeConversion  OutDataTypeStr=uint8  RndMeth=Round
  CAN1_CCU_AutoLampSts : Outport
  wires:
  Data Type Conversion/1 -> CAN1_CCU_AutoLampSts/1
  CCUAutoLampSts/1 -> Data Type Conversion/1

== system halout/HAL_OUT/CAN1/FD1_THCM1_0x182/CCUAutoMidLampSts ==
  CCUAutoMidLampSts : Inport
  Data Type Conversion : DataTypeConversion  OutDataTypeStr=uint8  RndMeth=Round
  CAN1_CCU_AutoMidLampSts : Outport
  wires:
  Data Type Conversion/1 -> CAN1_CCU_AutoMidLampSts/1
  CCUAutoMidLampSts/1 -> Data Type Conversion/1

== system halout/HAL_OUT/CAN1/FD1_THCM1_0x182/CCUDispalyRequest ==
  CCUDispalyRequest : Inport
  Data Type Conversion : DataTypeConversion  OutDataTypeStr=uint8  RndMeth=Round
  CAN1_CCU_Dispaly_Request : Outport
  wires:
  Data Type Conversion/1 -> CAN1_CCU_Dispaly_Request/1
  CCUDispalyRequest/1 -> Data Type Conversion/1

== system halout/HAL_OUT/CAN1/FD1_THCM1_0x182/CCUEcoSts ==
  CCUEcoSts : Inport
  Data Type Conversion : DataTypeConversion  OutDataTypeStr=uint8  RndMeth=Round
  CAN1_CCU_EcoSts : Outport
  wires:
  Data Type Conversion/1 -> CAN1_CCU_EcoSts/1
  CCUEcoSts/1 -> Data Type Conversion/1

== system halout/HAL_OUT/CAN1/FD1_THCM1_0x182/CCUFrtOnOffLampSts ==
  CCUFrtOnOffLampSts : Inport
  Data Type Conversion : DataTypeConversion  OutDataTypeStr=uint8  RndMeth=Round
  CAN1_CCU_FrtOnOffLampSts : Outport
  wires:
  Data Type Conversion/1 -> CAN1_CCU_FrtOnOffLampSts/1
  CCUFrtOnOffLampSts/1 -> Data Type Conversion/1

== system halout/HAL_OUT/CAN1/FD1_THCM1_0x182/CCUHEATMaxLampSts ==
  CCUHEATMaxLampSts : Inport
  Data Type Conversion : DataTypeConversion  OutDataTypeStr=uint8  RndMeth=Round
  CAN1_CCU_HEATMaxLampSts : Outport
  wires:
  Data Type Conversion/1 -> CAN1_CCU_HEATMaxLampSts/1
  CCUHEATMaxLampSts/1 -> Data Type Conversion/1

== system halout/HAL_OUT/CAN1/FD1_THCM1_0x182/CCURrOnOffLampSts ==
  CCURrOnOffLampSts : Inport
  Data Type Conversion : DataTypeConversion  OutDataTypeStr=uint8  RndMeth=Round
  CAN1_CCU_RrOnOffLampSts : Outport
  wires:
  Data Type Conversion/1 -> CAN1_CCU_RrOnOffLampSts/1
  CCURrOnOffLampSts/1 -> Data Type Conversion/1

== system halout/HAL_OUT/CAN1/FD1_THCM1_0x182/CCUSyncLampSts ==
  CCUSyncLampSts : Inport
  Data Type Conversion : DataTypeConversion  OutDataTypeStr=uint8  RndMeth=Round
  CAN1_CCU_SyncLampSts : Outport
  wires:
  Data Type Conversion/1 -> CAN1_CCU_SyncLampSts/1
  CCUSyncLampSts/1 -> Data Type Conversion/1

== system halout/HAL_OUT/CAN1/FD1_THCM1_0x182/CabinMode ==
  CabinMode : Inport
  Data Type Conversion : DataTypeConversion  OutDataTypeStr=uint8  RndMeth=Round
  CAN1_CabinMode : Outport
  wires:
  Data Type Conversion/1 -> CAN1_CabinMode/1
  CabinMode/1 -> Data Type Conversion/1

== system halout/HAL_OUT/CAN1/FD1_THCM1_0x182/EDriveMode ==
  EDriveMode : Inport
  Data Type Conversion : DataTypeConversion  OutDataTypeStr=uint8  RndMeth=Round
  CAN1_EDriveMode : Outport
  wires:
  Data Type Conversion/1 -> CAN1_EDriveMode/1
  EDriveMode/1 -> Data Type Conversion/1

== system halout/HAL_OUT/CAN1/FD1_THCM1_0x182/FDAGSCmd ==
  FDAGSCmd : Inport
  Data Type Conversion : DataTypeConversion  OutDataTypeStr=uint8  RndMeth=Round
  CAN1_FD_AGS_Cmd : Outport
  wires:
  Data Type Conversion/1 -> CAN1_FD_AGS_Cmd/1
  FDAGSCmd/1 -> Data Type Conversion/1

== system halout/HAL_OUT/CAN1/FD1_THCM1_0x182/FDRecyAutoCmd ==
  FDRecyAutoCmd : Inport
  Data Type Conversion : DataTypeConversion  OutDataTypeStr=uint8  RndMeth=Round
  CAN1_FD_RecyAuto_Cmd : Outport
  wires:
  Data Type Conversion/1 -> CAN1_FD_RecyAuto_Cmd/1
  FDRecyAutoCmd/1 -> Data Type Conversion/1

== system halout/HAL_OUT/CAN1/FD1_THCM1_0x182/FrCoolantflow ==
  FrCoolantflow : Inport
  Data Type Conversion : DataTypeConversion  OutDataTypeStr=uint8  RndMeth=Round
  convert_out : FVT_lib/hal/convert_out  gain=0.25  offset=0
  CAN1_Fr_Coolantflow : Outport
  wires:
  Data Type Conversion/1 -> CAN1_Fr_Coolantflow/1
  convert_out/1 -> Data Type Conversion/1
  FrCoolantflow/1 -> convert_out/1

== system halout/HAL_OUT/CAN1/FD1_THCM1_0x182/FrCoolanttemp ==
  FrCoolanttemp : Inport
  Data Type Conversion : DataTypeConversion  OutDataTypeStr=uint16  RndMeth=Round
  convert_out : FVT_lib/hal/convert_out  gain=1  offset=-40
  CAN1_Fr_Coolanttemp : Outport
  wires:
  Data Type Conversion/1 -> CAN1_Fr_Coolanttemp/1
  convert_out/1 -> Data Type Conversion/1
  FrCoolanttemp/1 -> convert_out/1

== system halout/HAL_OUT/CAN1/FD1_THCM1_0x182/HPThermalRecoveryReq ==
  HPThermalRecoveryReq : Inport
  Data Type Conversion : DataTypeConversion  OutDataTypeStr=uint8  RndMeth=Round
  CAN1_HPThermalRecoveryReq : Outport
  wires:
  Data Type Conversion/1 -> CAN1_HPThermalRecoveryReq/1
  HPThermalRecoveryReq/1 -> Data Type Conversion/1

== system halout/HAL_OUT/CAN1/FD1_THCM1_0x182/RrCoolantflow ==
  RrCoolantflow : Inport
  Data Type Conversion : DataTypeConversion  OutDataTypeStr=uint8  RndMeth=Round
  convert_out : FVT_lib/hal/convert_out  gain=0.25  offset=0
  CAN1_Rr_Coolantflow : Outport
  wires:
  Data Type Conversion/1 -> CAN1_Rr_Coolantflow/1
  convert_out/1 -> Data Type Conversion/1
  RrCoolantflow/1 -> convert_out/1

== system halout/HAL_OUT/CAN1/FD1_THCM1_0x182/RrCoolanttemp ==
  RrCoolanttemp : Inport
  Data Type Conversion : DataTypeConversion  OutDataTypeStr=uint16  RndMeth=Round
  convert_out : FVT_lib/hal/convert_out  gain=1  offset=-40
  CAN1_Rr_Coolanttemp : Outport
  wires:
  Data Type Conversion/1 -> CAN1_Rr_Coolanttemp/1
  convert_out/1 -> Data Type Conversion/1
  RrCoolanttemp/1 -> convert_out/1

== system halout/HAL_OUT/CAN1/FD1_THCM1_0x182/sigAirIntenZon1St ==
  sigAirIntenZon1St : Inport
  Data Type Conversion : DataTypeConversion  OutDataTypeStr=uint8  RndMeth=Round
  CAN1_sigAirIntenZon1St : Outport
  wires:
  Data Type Conversion/1 -> CAN1_sigAirIntenZon1St/1
  sigAirIntenZon1St/1 -> Data Type Conversion/1

== system halout/HAL_OUT/CAN1/FD1_THCM1_0x182/sigAirIntenZon3St ==
  sigAirIntenZon3St : Inport
  Data Type Conversion : DataTypeConversion  OutDataTypeStr=uint8  RndMeth=Round
  CAN1_sigAirIntenZon3St : Outport
  wires:
  Data Type Conversion/1 -> CAN1_sigAirIntenZon3St/1
  sigAirIntenZon3St/1 -> Data Type Conversion/1

== system halout/HAL_OUT/CAN1/FD1_THCM1_0x182/sigAmbAirT ==
  sigAmbAirT : Inport
  Data Type Conversion : DataTypeConversion  OutDataTypeStr=uint8  RndMeth=Round
  convert_out : FVT_lib/hal/convert_out  gain=0.5  offset=-40
  CAN1_sigAmbAirT : Outport
  wires:
  Data Type Conversion/1 -> CAN1_sigAmbAirT/1
  convert_out/1 -> Data Type Conversion/1
  sigAmbAirT/1 -> convert_out/1

== system halout/HAL_OUT/CAN1/FD1_THCM1_0x182/sigCbnAirT ==
  sigCbnAirT : Inport
  Data Type Conversion : DataTypeConversion  OutDataTypeStr=uint8  RndMeth=Round
  convert_out : FVT_lib/hal/convert_out  gain=0.5  offset=-40
  CAN1_sigCbnAirT : Outport
  wires:
  Data Type Conversion/1 -> CAN1_sigCbnAirT/1
  convert_out/1 -> Data Type Conversion/1
  sigCbnAirT/1 -> convert_out/1

== system halout/HAL_OUT/CAN1/FD1_THCM1_0x182/sigCbnPTCPwrAct ==
  sigCbnPTCPwrAct : Inport
  Data Type Conversion : DataTypeConversion  OutDataTypeStr=uint8  RndMeth=Round
  convert_out : FVT_lib/hal/convert_out  gain=50  offset=0
  CAN1_sigCbnPTCPwrAct : Outport
  wires:
  Data Type Conversion/1 -> CAN1_sigCbnPTCPwrAct/1
  convert_out/1 -> Data Type Conversion/1
  sigCbnPTCPwrAct/1 -> convert_out/1

== system halout/HAL_OUT/CAN1/FD1_THCM1_0x182/sigCbnSolarLeft ==
  sigCbnSolarLeft : Inport
  Data Type Conversion : DataTypeConversion  OutDataTypeStr=uint8  RndMeth=Round
  convert_out : FVT_lib/hal/convert_out  gain=5  offset=0
  CAN1_sigCbnSolarLeft : Outport
  wires:
  Data Type Conversion/1 -> CAN1_sigCbnSolarLeft/1
  convert_out/1 -> Data Type Conversion/1
  sigCbnSolarLeft/1 -> convert_out/1

== system halout/HAL_OUT/CAN1/FD1_THCM1_0x182/sigCbnSolarRight ==
  sigCbnSolarRight : Inport
  Data Type Conversion : DataTypeConversion  OutDataTypeStr=uint8  RndMeth=Round
  convert_out : FVT_lib/hal/convert_out  gain=5  offset=0
  CAN1_sigCbnSolarRight : Outport
  wires:
  Data Type Conversion/1 -> CAN1_sigCbnSolarRight/1
  convert_out/1 -> Data Type Conversion/1
  sigCbnSolarRight/1 -> convert_out/1

== system halout/HAL_OUT/CAN1/FD1_THCM1_0x182/sigClmtCmprPwrAct ==
  sigClmtCmprPwrAct : Inport
  Data Type Conversion : DataTypeConversion  OutDataTypeStr=uint8  RndMeth=Round
  convert_out : FVT_lib/hal/convert_out  gain=50  offset=0
  CAN1_sigClmtCmprPwrAct : Outport
  wires:
  Data Type Conversion/1 -> CAN1_sigClmtCmprPwrAct/1
  convert_out/1 -> Data Type Conversion/1
  sigClmtCmprPwrAct/1 -> convert_out/1

== system halout/HAL_OUT/CAN1/FD1_THCM1_0x182/sigClntTHvBattOut ==
  sigClntTHvBattOut : Inport
  Data Type Conversion : DataTypeConversion  OutDataTypeStr=uint8  RndMeth=Round
  convert_out : FVT_lib/hal/convert_out  gain=0.5  offset=-40
  CAN1_sigClntTHvBattOut : Outport
  wires:
  Data Type Conversion/1 -> CAN1_sigClntTHvBattOut/1
  convert_out/1 -> Data Type Conversion/1
  sigClntTHvBattOut/1 -> convert_out/1

== system halout/HAL_OUT/CAN1/FD1_THCM1_0x182/sigDfrstSt ==
  sigDfrstSt : Inport
  Data Type Conversion : DataTypeConversion  OutDataTypeStr=uint8  RndMeth=Round
  CAN1_sigDfrstSt : Outport
  wires:
  Data Type Conversion/1 -> CAN1_sigDfrstSt/1
  sigDfrstSt/1 -> Data Type Conversion/1

== system halout/HAL_OUT/CAN1/FD1_THCM1_0x182/sigHvacSt ==
  sigHvacSt : Inport
  Data Type Conversion : DataTypeConversion  OutDataTypeStr=uint8  RndMeth=Round
  CAN1_sigHvacSt : Outport
  wires:
  Data Type Conversion/1 -> CAN1_sigHvacSt/1
  sigHvacSt/1 -> Data Type Conversion/1

== system halout/HAL_OUT/CAN1/FD1_THCM1_0x182/sigRecircSt ==
  sigRecircSt : Inport
  Data Type Conversion : DataTypeConversion  OutDataTypeStr=uint8  RndMeth=Round
  CAN1_sigRecircSt : Outport
  wires:
  Data Type Conversion/1 -> CAN1_sigRecircSt/1
  sigRecircSt/1 -> Data Type Conversion/1

== system halout/HAL_OUT/CAN1/FD1_THCM1_0x182/sigSetTempZon1St ==
  sigSetTempZon1St : Inport
  Data Type Conversion : DataTypeConversion  OutDataTypeStr=uint8  RndMeth=Round
  convert_out : FVT_lib/hal/convert_out  gain=0.5  offset=17
  CAN1_sigSetTempZon1St : Outport
  wires:
  Data Type Conversion/1 -> CAN1_sigSetTempZon1St/1
  convert_out/1 -> Data Type Conversion/1
  sigSetTempZon1St/1 -> convert_out/1

== system halout/HAL_OUT/CAN1/FD1_THCM1_0x182/sigSetTempZon2St ==
  sigSetTempZon2St : Inport
  Data Type Conversion : DataTypeConversion  OutDataTypeStr=uint8  RndMeth=Round
  convert_out : FVT_lib/hal/convert_out  gain=0.5  offset=17
  CAN1_sigSetTempZon2St : Outport
  wires:
  Data Type Conversion/1 -> CAN1_sigSetTempZon2St/1
  convert_out/1 -> Data Type Conversion/1
  sigSetTempZon2St/1 -> convert_out/1

== system halout/HAL_OUT/CAN1/FD1_THCM1_0x182/sigSetTempZon3St ==
  sigSetTempZon3St : Inport
  Data Type Conversion : DataTypeConversion  OutDataTypeStr=uint8  RndMeth=Round
  convert_out : FVT_lib/hal/convert_out  gain=0.5  offset=17
  CAN1_sigSetTempZon3St : Outport
  wires:
  Data Type Conversion/1 -> CAN1_sigSetTempZon3St/1
  convert_out/1 -> Data Type Conversion/1
  sigSetTempZon3St/1 -> convert_out/1

== system halout/HAL_OUT/CAN1/FD1_THCM1_0x182/sigWindDirZon1St ==
  sigWindDirZon1St : Inport
  Data Type Conversion : DataTypeConversion  OutDataTypeStr=uint8  RndMeth=Round
  CAN1_sigWindDirZon1St : Outport
  wires:
  Data Type Conversion/1 -> CAN1_sigWindDirZon1St/1
  sigWindDirZon1St/1 -> Data Type Conversion/1

== system halout/HAL_OUT/CAN1/FD1_THCM1_0x182/sigWindDirZon3St ==
  sigWindDirZon3St : Inport
  Data Type Conversion : DataTypeConversion  OutDataTypeStr=uint8  RndMeth=Round
  CAN1_sigWindDirZon3St : Outport
  wires:
  Data Type Conversion/1 -> CAN1_sigWindDirZon3St/1
  sigWindDirZon3St/1 -> Data Type Conversion/1

== system halout/HAL_OUT/CAN1/FD1_VCU1_0x116/CCCrlSta ==
  CCCrlSta : Inport
  Data Type Conversion : DataTypeConversion  OutDataTypeStr=uint8  RndMeth=Round
  CAN1_CC_Crl_Sta : Outport
  wires:
  Data Type Conversion/1 -> CAN1_CC_Crl_Sta/1
  CCCrlSta/1 -> Data Type Conversion/1

== system halout/HAL_OUT/CAN1/FD1_VCU1_0x116/EngAGSCloseSta ==
  EngAGSCloseSta : Inport
  Data Type Conversion : DataTypeConversion  OutDataTypeStr=uint8  RndMeth=Round
  CAN1_Eng_AGSCloseSta : Outport
  wires:
  Data Type Conversion/1 -> CAN1_Eng_AGSCloseSta/1
  EngAGSCloseSta/1 -> Data Type Conversion/1

== system halout/HAL_OUT/CAN1/FD1_VCU1_0x116/EngActvDmpDisabSta ==
  EngActvDmpDisabSta : Inport
  Data Type Conversion : DataTypeConversion  OutDataTypeStr=uint8  RndMeth=Round
  CAN1_Eng_ActvDmpDisabSta : Outport
  wires:
  Data Type Conversion/1 -> CAN1_Eng_ActvDmpDisabSta/1
  EngActvDmpDisabSta/1 -> Data Type Conversion/1

== system halout/HAL_OUT/CAN1/FD1_VCU1_0x116/EngCoastDwSta ==
  EngCoastDwSta : Inport
  Data Type Conversion : DataTypeConversion  OutDataTypeStr=uint8  RndMeth=Round
  CAN1_Eng_CoastDwSta : Outport
  wires:
  Data Type Conversion/1 -> CAN1_Eng_CoastDwSta/1
  EngCoastDwSta/1 -> Data Type Conversion/1

== system halout/HAL_OUT/CAN1/FD1_VCU1_0x116/EngPwrLockSta ==
  EngPwrLockSta : Inport
  Data Type Conversion : DataTypeConversion  OutDataTypeStr=uint8  RndMeth=Round
  CAN1_Eng_PwrLockSta : Outport
  wires:
  Data Type Conversion/1 -> CAN1_Eng_PwrLockSta/1
  EngPwrLockSta/1 -> Data Type Conversion/1

== system halout/HAL_OUT/CAN1/FD1_VCU1_0x116/HVPwrSta ==
  HVPwrSta : Inport
  Data Type Conversion : DataTypeConversion  OutDataTypeStr=uint8  RndMeth=Round
  CAN1_HVPwrSta : Outport
  wires:
  Data Type Conversion/1 -> CAN1_HVPwrSta/1
  HVPwrSta/1 -> Data Type Conversion/1

== system halout/HAL_OUT/CAN1/FD1_VCU1_0x116/LVPwrSta ==
  LVPwrSta : Inport
  Data Type Conversion : DataTypeConversion  OutDataTypeStr=uint8  RndMeth=Round
  CAN1_LVPwrSta : Outport
  wires:
  Data Type Conversion/1 -> CAN1_LVPwrSta/1
  LVPwrSta/1 -> Data Type Conversion/1

== system halout/HAL_OUT/CAN1/FD1_VCU1_0x116/MSACrlSta ==
  MSACrlSta : Inport
  Data Type Conversion : DataTypeConversion  OutDataTypeStr=uint8  RndMeth=Round
  CAN1_MSA_Crl_Sta : Outport
  wires:
  Data Type Conversion/1 -> CAN1_MSA_Crl_Sta/1
  MSACrlSta/1 -> Data Type Conversion/1

== system halout/HAL_OUT/CAN1/FD1_VCU1_0x116/PButtonSta ==
  PButtonSta : Inport
  Data Type Conversion : DataTypeConversion  OutDataTypeStr=uint8  RndMeth=Round
  CAN1_P_Button_Sta : Outport
  wires:
  Data Type Conversion/1 -> CAN1_P_Button_Sta/1
  PButtonSta/1 -> Data Type Conversion/1

== system halout/HAL_OUT/CAN1/FD1_VCU1_0x116/PrkReq ==
  PrkReq : Inport
  Data Type Conversion : DataTypeConversion  OutDataTypeStr=uint8  RndMeth=Round
  CAN1_PrkReq : Outport
  wires:
  Data Type Conversion/1 -> CAN1_PrkReq/1
  PrkReq/1 -> Data Type Conversion/1

== system halout/HAL_OUT/CAN1/FD1_VCU1_0x116/PrkReqValid ==
  PrkReqValid : Inport
  Data Type Conversion : DataTypeConversion  OutDataTypeStr=uint8  RndMeth=Round
  CAN1_PrkReqValid : Outport
  wires:
  Data Type Conversion/1 -> CAN1_PrkReqValid/1
  PrkReqValid/1 -> Data Type Conversion/1

== system halout/HAL_OUT/CAN1/FD1_VCU1_0x116/PwrSta ==
  PwrSta : Inport
  Data Type Conversion : DataTypeConversion  OutDataTypeStr=uint8  RndMeth=Round
  CAN1_PwrSta : Outport
  wires:
  Data Type Conversion/1 -> CAN1_PwrSta/1
  PwrSta/1 -> Data Type Conversion/1

== system halout/HAL_OUT/CAN1/FD1_VCU1_0x116/ShiftGearPosn ==
  ShiftGearPosn : Inport
  Data Type Conversion : DataTypeConversion  OutDataTypeStr=uint8  RndMeth=Round
  CAN1_ShiftGearPosn : Outport
  wires:
  Data Type Conversion/1 -> CAN1_ShiftGearPosn/1
  ShiftGearPosn/1 -> Data Type Conversion/1

== system halout/HAL_OUT/CAN1/FD1_VCU1_0x116/VehMalfunLevel ==
  VehMalfunLevel : Inport
  Data Type Conversion : DataTypeConversion  OutDataTypeStr=uint8  RndMeth=Round
  CAN1_VehMalfunLevel : Outport
  wires:
  Data Type Conversion/1 -> CAN1_VehMalfunLevel/1
  VehMalfunLevel/1 -> Data Type Conversion/1

== system halout/HAL_OUT/CAN1/FD1_VCU1_0x116/XWDMode ==
  XWDMode : Inport
  Data Type Conversion : DataTypeConversion  OutDataTypeStr=uint8  RndMeth=Round
  CAN1_XWDMode : Outport
  wires:
  Data Type Conversion/1 -> CAN1_XWDMode/1
  XWDMode/1 -> Data Type Conversion/1

== system halout/HAL_OUT/CAN1/FD1_VCU2_0x154/ACCCtrlAvail ==
  ACCCtrlAvail : Inport
  Data Type Conversion : DataTypeConversion  OutDataTypeStr=uint8  RndMeth=Round
  CAN1_ACC_CtrlAvail : Outport
  wires:
  Data Type Conversion/1 -> CAN1_ACC_CtrlAvail/1
  ACCCtrlAvail/1 -> Data Type Conversion/1

== system halout/HAL_OUT/CAN1/FD1_VCU2_0x154/AccPedalOverride ==
  AccPedalOverride : Inport
  Data Type Conversion : DataTypeConversion  OutDataTypeStr=uint8  RndMeth=Round
  CAN1_AccPedal_Override : Outport
  wires:
  Data Type Conversion/1 -> CAN1_AccPedal_Override/1
  AccPedalOverride/1 -> Data Type Conversion/1

== system halout/HAL_OUT/CAN1/FD1_VCU2_0x154/ActAPSPosn ==
  ActAPSPosn : Inport
  Data Type Conversion : DataTypeConversion  OutDataTypeStr=uint8  RndMeth=Round
  convert_out : FVT_lib/hal/convert_out  gain=0.394  offset=0
  CAN1_ActAPSPosn : Outport
  wires:
  Data Type Conversion/1 -> CAN1_ActAPSPosn/1
  convert_out/1 -> Data Type Conversion/1
  ActAPSPosn/1 -> convert_out/1

== system halout/HAL_OUT/CAN1/FD1_VCU2_0x154/Byte_0 ==
  CS_VCU2_CAN1 : Inport
  BitwiseOR : simulink/Logic and Bit Operations/Bitwise Operator  logicop=OR  UseBitMask=off  BitMask=bin2dec('11011001')  BitMaskRealWorld=Stored Integer
  SignalPack : FVT_lib/hal/SignalPack  RightShiftCnt=0  BitMask=2^8-1  LeftShiftCnt=0
  UnitConverter : DataTypeConversion  OutDataTypeStr=uint8  RndMeth=Round
  UnitConverter1 : DataTypeConversion  OutDataTypeStr=uint8  RndMeth=Round
  Byte_0 : Outport
  wires:
  BitwiseOR/1 -> Byte_0/1
  UnitConverter/1 -> BitwiseOR/1
  SignalPack/1 -> UnitConverter/1
  UnitConverter1/1 -> SignalPack/1
  CS_VCU2_CAN1/1 -> UnitConverter1/1

== system halout/HAL_OUT/CAN1/FD1_VCU2_0x154/Byte_1 ==
  RC_VCU2_CAN1 : Inport
  BitwiseOR : simulink/Logic and Bit Operations/Bitwise Operator  logicop=OR  UseBitMask=off  BitMask=bin2dec('11011001')  BitMaskRealWorld=Stored Integer
  SignalPack : FVT_lib/hal/SignalPack  RightShiftCnt=0  BitMask=2^4-1  LeftShiftCnt=0
  UnitConverter : DataTypeConversion  OutDataTypeStr=uint8  RndMeth=Round
  UnitConverter1 : DataTypeConversion  OutDataTypeStr=uint8  RndMeth=Round
  Byte_1 : Outport
  wires:
  BitwiseOR/1 -> Byte_1/1
  UnitConverter/1 -> BitwiseOR/1
  SignalPack/1 -> UnitConverter/1
  UnitConverter1/1 -> SignalPack/1
  RC_VCU2_CAN1/1 -> UnitConverter1/1

== system halout/HAL_OUT/CAN1/FD1_VCU2_0x154/Byte_10 ==
  VehActPwr : Inport
  BitwiseOR : simulink/Logic and Bit Operations/Bitwise Operator  logicop=OR  UseBitMask=off  BitMask=bin2dec('11011001')  BitMaskRealWorld=Stored Integer
  SignalPack : FVT_lib/hal/SignalPack  RightShiftCnt=16  BitMask=2^8-1  LeftShiftCnt=0
  UnitConverter : DataTypeConversion  OutDataTypeStr=uint8  RndMeth=Round
  UnitConverter1 : DataTypeConversion  OutDataTypeStr=uint32  RndMeth=Round
  convert_out : FVT_lib/hal/convert_out  gain=1  offset=-600000
  Byte_10 : Outport
  wires:
  BitwiseOR/1 -> Byte_10/1
  UnitConverter/1 -> BitwiseOR/1
  SignalPack/1 -> UnitConverter/1
  UnitConverter1/1 -> SignalPack/1
  convert_out/1 -> UnitConverter1/1
  VehActPwr/1 -> convert_out/1

== system halout/HAL_OUT/CAN1/FD1_VCU2_0x154/Byte_11 ==
  VehActPwr : Inport
  BitwiseOR : simulink/Logic and Bit Operations/Bitwise Operator  logicop=OR  UseBitMask=off  BitMask=bin2dec('11011001')  BitMaskRealWorld=Stored Integer
  SignalPack : FVT_lib/hal/SignalPack  RightShiftCnt=8  BitMask=2^8-1  LeftShiftCnt=0
  UnitConverter : DataTypeConversion  OutDataTypeStr=uint8  RndMeth=Round
  UnitConverter1 : DataTypeConversion  OutDataTypeStr=uint32  RndMeth=Round
  convert_out : FVT_lib/hal/convert_out  gain=1  offset=-600000
  Byte_11 : Outport
  wires:
  BitwiseOR/1 -> Byte_11/1
  UnitConverter/1 -> BitwiseOR/1
  SignalPack/1 -> UnitConverter/1
  UnitConverter1/1 -> SignalPack/1
  convert_out/1 -> UnitConverter1/1
  VehActPwr/1 -> convert_out/1

== system halout/HAL_OUT/CAN1/FD1_VCU2_0x154/Byte_12 ==
  VehActPwr : Inport
  BitwiseOR : simulink/Logic and Bit Operations/Bitwise Operator  logicop=OR  UseBitMask=off  BitMask=bin2dec('11011001')  BitMaskRealWorld=Stored Integer
  SignalPack : FVT_lib/hal/SignalPack  RightShiftCnt=0  BitMask=2^8-1  LeftShiftCnt=0
  UnitConverter : DataTypeConversion  OutDataTypeStr=uint8  RndMeth=Round
  UnitConverter1 : DataTypeConversion  OutDataTypeStr=uint32  RndMeth=Round
  convert_out : FVT_lib/hal/convert_out  gain=1  offset=-600000
  Byte_12 : Outport
  wires:
  BitwiseOR/1 -> Byte_12/1
  UnitConverter/1 -> BitwiseOR/1
  SignalPack/1 -> UnitConverter/1
  UnitConverter1/1 -> SignalPack/1
  convert_out/1 -> UnitConverter1/1
  VehActPwr/1 -> convert_out/1

== system halout/HAL_OUT/CAN1/FD1_VCU2_0x154/Byte_13 ==
  DriverTq : Inport
  BitwiseOR : simulink/Logic and Bit Operations/Bitwise Operator  logicop=OR  UseBitMask=off  BitMask=bin2dec('11011001')  BitMaskRealWorld=Stored Integer
  SignalPack : FVT_lib/hal/SignalPack  RightShiftCnt=8  BitMask=2^8-1  LeftShiftCnt=0
  UnitConverter : DataTypeConversion  OutDataTypeStr=uint8  RndMeth=Round
  UnitConverter1 : DataTypeConversion  OutDataTypeStr=uint16  RndMeth=Round
  convert_out : FVT_lib/hal/convert_out  gain=1  offset=-4300
  Byte_13 : Outport
  wires:
  BitwiseOR/1 -> Byte_13/1
  UnitConverter/1 -> BitwiseOR/1
  SignalPack/1 -> UnitConverter/1
  UnitConverter1/1 -> SignalPack/1
  convert_out/1 -> UnitConverter1/1
  DriverTq/1 -> convert_out/1

== system halout/HAL_OUT/CAN1/FD1_VCU2_0x154/Byte_14 ==
  DriverTq : Inport
  BitwiseOR : simulink/Logic and Bit Operations/Bitwise Operator  logicop=OR  UseBitMask=off  BitMask=bin2dec('11011001')  BitMaskRealWorld=Stored Integer
  SignalPack : FVT_lib/hal/SignalPack  RightShiftCnt=0  BitMask=2^8-1  LeftShiftCnt=0
  UnitConverter : DataTypeConversion  OutDataTypeStr=uint8  RndMeth=Round
  UnitConverter1 : DataTypeConversion  OutDataTypeStr=uint16  RndMeth=Round
  convert_out : FVT_lib/hal/convert_out  gain=1  offset=-4300
  Byte_14 : Outport
  wires:
  BitwiseOR/1 -> Byte_14/1
  UnitConverter/1 -> BitwiseOR/1
  SignalPack/1 -> UnitConverter/1
  UnitConverter1/1 -> SignalPack/1
  convert_out/1 -> UnitConverter1/1
  DriverTq/1 -> convert_out/1

== system halout/HAL_OUT/CAN1/FD1_VCU2_0x154/Byte_15 ==
  ActAPSPosn : Inport
  BitwiseOR : simulink/Logic and Bit Operations/Bitwise Operator  logicop=OR  UseBitMask=off  BitMask=bin2dec('11011001')  BitMaskRealWorld=Stored Integer
  SignalPack : FVT_lib/hal/SignalPack  RightShiftCnt=0  BitMask=2^8-1  LeftShiftCnt=0
  UnitConverter : DataTypeConversion  OutDataTypeStr=uint8  RndMeth=Round
  UnitConverter1 : DataTypeConversion  OutDataTypeStr=uint8  RndMeth=Round
  convert_out : FVT_lib/hal/convert_out  gain=0.394  offset=0
  Byte_15 : Outport
  wires:
  BitwiseOR/1 -> Byte_15/1
  UnitConverter/1 -> BitwiseOR/1
  SignalPack/1 -> UnitConverter/1
  UnitConverter1/1 -> SignalPack/1
  convert_out/1 -> UnitConverter1/1
  ActAPSPosn/1 -> convert_out/1

== system halout/HAL_OUT/CAN1/FD1_VCU2_0x154/Byte_2 ==
  Fr_DriverTq : Inport
  BitwiseOR : simulink/Logic and Bit Operations/Bitwise Operator  logicop=OR  UseBitMask=off  BitMask=bin2dec('11011001')  BitMaskRealWorld=Stored Integer
  SignalPack : FVT_lib/hal/SignalPack  RightShiftCnt=8  BitMask=2^8-1  LeftShiftCnt=0
  UnitConverter : DataTypeConversion  OutDataTypeStr=uint8  RndMeth=Round
  UnitConverter1 : DataTypeConversion  OutDataTypeStr=uint16  RndMeth=Round
  convert_out : FVT_lib/hal/convert_out  gain=0.5  offset=-5300
  Byte_2 : Outport
  wires:
  BitwiseOR/1 -> Byte_2/1
  UnitConverter/1 -> BitwiseOR/1
  SignalPack/1 -> UnitConverter/1
  UnitConverter1/1 -> SignalPack/1
  convert_out/1 -> UnitConverter1/1
  Fr_DriverTq/1 -> convert_out/1
